simulink model "CheckFingerFunction"  (R2024a)
settings: Solver=VariableStepAuto  StartTime=0.0  StopTime=0.32  FixedStep=0.001  MaxStep=0.05  RelTol=1e-3
values from neighbouring files (symbols this model uses):
  CollisionOpacity = 0.1    [InitTestParams.m]
  g = 9.81    [InitTestParams.m]
  MotorTorque = 0.4    [InitTestParams.m]
undefined symbols (not defined in the file or in its folder): Ball, S1, S2, S3, X, Y, Z
libraries: sm_lib x404, nesl_utility x200
(part 2 of 8)

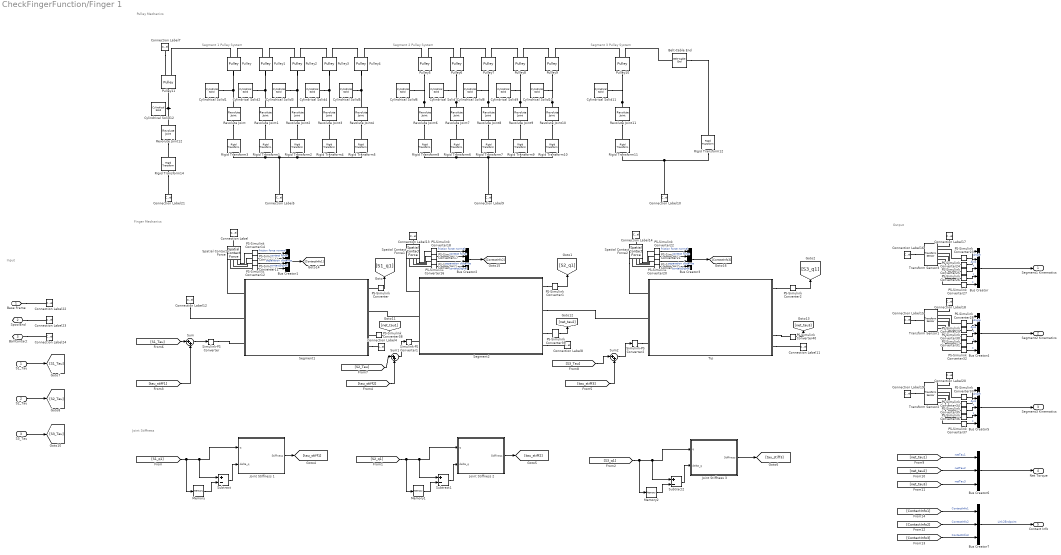
== system CheckFingerFunction/Finger 1 ==
  note: Output
  note: Input
  note: Pulley Mechanics
  note: Finger Mechanics
  note: Joint Stiffness
  note: Segment 1 Pulley System
  note: Segment 2 Pulley System
  note: Segment 3 Pulley System
  S1_Tau : Inport
  S2_Tau : Inport  Port=2
  S3_Tau : Inport  Port=3
  Belt-Cable End : sm_lib/Belts and Cables/Belt-Cable End
  Bus Creator : BusCreator  Inputs=5
  Bus Creator1 : BusCreator  Inputs=4
  Bus Creator2 : BusCreator  Inputs=4
  Bus Creator3 : BusCreator  Inputs=4
  Bus Creator4 : BusCreator  Inputs=5
  Bus Creator5 : BusCreator  Inputs=5
  Bus Creator6 : BusCreator  Inputs=3
  Bus Creator7 : BusCreator  Inputs=3
  Connection Label{,13..14,24} (4 alike) : ConnectionLabel  Label=BallContact
  Connection Label10 : ConnectionLabel  Label=PulleyFrame3
  Connection Label11 : ConnectionLabel  Label=PulleyFrame3
  Connection Label{12,15..16,19,21..22} (6 alike) : ConnectionLabel  Label=BaseFrame
  Connection Label17 : ConnectionLabel  Label=PulleyFrame1
  Connection Label18 : ConnectionLabel  Label=PulleyFrame2
  Connection Label20 : ConnectionLabel  Label=PulleyFrame3
  Connection Label23 : ConnectionLabel  Label=SpoolEnd
  Connection Label4 : ConnectionLabel  Label=PulleyFrame1
  Connection Label5 : ConnectionLabel  Label=PulleyFrame1
  Connection Label7 : ConnectionLabel  Label=SpoolEnd
  Connection Label8 : ConnectionLabel  Label=PulleyFrame2
  Connection Label9 : ConnectionLabel  Label=PulleyFrame2
  Cylindrical Solid{1..12} (12 alike) : sm_lib/Body Elements/Cylindrical Solid  CylinderRadius=1  CylinderRadiusUnits=mm  CylinderLength=1  CylinderLengthUnits=mm  ExportEntireGeometry=off  InertiaType=CalculateFromGeometry  BasedOnType=Density  Density=1000  DensityUnits=kg/m^3  Mass=1  MassUnits=kg  CenterOfMass=[0 0 0]  CenterOfMassUnits=m  MomentsOfInertia=[1 1 1]  MomentsOfInertiaUnits=kg*m^2  ProductsOfInertia=[0 0 0]  ProductsOfInertiaUnits=kg*m^2  GraphicType=FromGeometry  MarkerShape=Sphere  MarkerSize=10  GraphicVisPropType=SimpleVisualProperties  GraphicDiffuseColor=[0.5 0.5 0.5]  GraphicOpacity=1.0  GraphicSpecularColor=[0.5 0.5 0.5 1.0]  GraphicAmbientColor=[0.15 0.15 0.15 1.0]  GraphicEmissiveColor=[0.0 0.0 0.0 1.0]  GraphicShininess=75  DoExposeReferenceFrame=on  SerializedFrames=<Frames/>
  Joint Stiffness 1 : MATLAB Function  TreatAsAtomicUnit=on  mask{tau_s=0, DynamicStiffness=0}
  Joint Stiffness 2 : MATLAB Function  TreatAsAtomicUnit=on  mask{tau_s=S2.tau_s, DynamicStiffness=S2.K}
  Joint Stiffness 3 : MATLAB Function  TreatAsAtomicUnit=on  mask{tau_s=S3.tau_s, DynamicStiffness=S3.K}
  Memory : Memory
  Memory1 : Memory
  Memory2 : Memory
  PS-Simulink Converter{,1..2,11..22,38..40} (18 alike) : nesl_utility/PS-Simulink Converter  PhysicalDomain=network_engine_domain  SubClassName=ps_output  LeftPortType=input  RightPortType=output  PseudoPeriodic=off  Frequencies=[]  VectorFormat=inherit  Unit=inherit  AffineConversion=off
  PS-Simulink Converter{23..37} (15 alike) : nesl_utility/PS-Simulink Converter  PhysicalDomain=network_engine_domain  SubClassName=ps_output  LeftPortType=input  RightPortType=output  PseudoPeriodic=off  Frequencies=[]  VectorFormat=1-D array  Unit=inherit  AffineConversion=off
  Pulley{,1..11} (12 alike) : sm_lib/Belts and Cables/Pulley  PitchRadius=0.001  PitchRadiusUnits=mm  InitialWrapAngleLowerBound=0.0  InitialWrapAngleLowerBoundUnits=deg  SenseWrapAngle=off  SensePulleyAngleA=off  SensePulleyAngleB=off  SenseFleetAngleA=off  SenseFleetAngleB=off
  Revolute Joint{,1..4,6..12} (12 alike) : sm_lib/Joints/Revolute Joint  JointMode=Normal  CompositeWrenchDir=FollowerOnBase  CompositeWrenchFrame=BaseFrame  SenseConstraintForce=off  SenseConstraintTorque=off  SenseTotalForce=off  SenseTotalTorque=off  PositionTargetSpecify=off  PositionTargetPriority=High  PositionTargetValue=0  PositionTargetValueUnits=deg  VelocityTargetSpecify=off  VelocityTargetPriority=High  VelocityTargetValue=0  VelocityTargetValueUnits=deg/s  EquilibriumPosition=0  EquilibriumPositionUnits=deg  SpringStiffness=0  SpringStiffnessUnits=N*m/deg  DampingCoefficient=0  DampingCoefficientUnits=N*m/(deg/s)  LowerLimitSpecify=off  LowerLimitBound=-90  LowerLimitBoundUnits=deg  LowerLimitStiffness=1e4  LowerLimitStiffnessUnits=N*m/deg  LowerLimitDamping=10  LowerLimitDampingUnits=N*m/(deg/s)  LowerLimitTransitionRegionWidth=0.1  LowerLimitTransitionRegionWidthUnits=deg  UpperLimitSpecify=off  UpperLimitBound=90  UpperLimitBoundUnits=deg  UpperLimitStiffness=1e4  UpperLimitStiffnessUnits=N*m/deg  UpperLimitDamping=10  UpperLimitDampingUnits=N*m/(deg/s)  UpperLimitTransitionRegionWidth=0.1  UpperLimitTransitionRegionWidthUnits=deg  TorqueActuationMode=NoTorque  MotionActuationMode=ComputedMotion  SensePosition=off  SenseVelocity=off  SenseAcceleration=off  SenseTorqueForce=off  SenseLowerLimitTorqueForce=off  SenseUpperLimitTorqueForce=off
  Rigid Transform1 : sm_lib/Frames and Transforms/Rigid Transform  RotationMethod=None  FollAlignAxisA=+Z  BaseAlignAxisA=+Z  FollAlignAxisB=+X  BaseAlignAxisB=+X  RotationStandardAxis=+Z  RotationAngle=0  RotationAngleUnits=deg  RotationArbitraryAxis=[0 0 1]  RotationSequenceAxes=FollowerAxes  RotationSequence=XYX  RotationSequenceAngles=[0 0 0]  RotationSequenceAnglesUnits=deg  RotationMatrix=[1 0 0; 0 1 0; 0 0 1]  Quaternion=[1 0 0 0]  TranslationMethod=Cartesian  TranslationCartesianOffset=[12.85 4 0]  TranslationCartesianOffsetUnits=mm  TranslationStandardAxis=+Z  TranslationStandardOffset=0  TranslationStandardOffsetUnits=mm  TranslationROffset=0  TranslationROffsetUnits=m  TranslationThetaOffset=0  TranslationThetaOffsetUnits=deg  TranslationZOffset=0  TranslationZOffsetUnits=m
  Rigid Transform10 : sm_lib/Frames and Transforms/Rigid Transform  RotationMethod=None  FollAlignAxisA=+Z  BaseAlignAxisA=-Z  FollAlignAxisB=+Y  BaseAlignAxisB=+Y  RotationStandardAxis=+Z  RotationAngle=0  RotationAngleUnits=deg  RotationArbitraryAxis=[0 0 1]  RotationSequenceAxes=FollowerAxes  RotationSequence=XYX  RotationSequenceAngles=[0 0 0]  RotationSequenceAnglesUnits=deg  RotationMatrix=[1 0 0; 0 1 0; 0 0 1]  Quaternion=[1 0 0 0]  TranslationMethod=Cartesian  TranslationCartesianOffset=[30 10 0]  TranslationCartesianOffsetUnits=mm  TranslationStandardAxis=+Z  TranslationStandardOffset=0  TranslationStandardOffsetUnits=mm  TranslationROffset=0  TranslationROffsetUnits=m  TranslationThetaOffset=0  TranslationThetaOffsetUnits=deg  TranslationZOffset=0  TranslationZOffsetUnits=m
  Rigid Transform11 : sm_lib/Frames and Transforms/Rigid Transform  RotationMethod=AlignedAxes  FollAlignAxisA=-Z  BaseAlignAxisA=+Z  FollAlignAxisB=+Y  BaseAlignAxisB=+Y  RotationStandardAxis=+Z  RotationAngle=0  RotationAngleUnits=deg  RotationArbitraryAxis=[0 0 1]  RotationSequenceAxes=FollowerAxes  RotationSequence=XYX  RotationSequenceAngles=[0 0 0]  RotationSequenceAnglesUnits=deg  RotationMatrix=[1 0 0; 0 1 0; 0 0 1]  Quaternion=[1 0 0 0]  TranslationMethod=Cartesian  TranslationCartesianOffset=[14.34 3.5 0]  TranslationCartesianOffsetUnits=mm  TranslationStandardAxis=+Z  TranslationStandardOffset=0  TranslationStandardOffsetUnits=mm  TranslationROffset=0  TranslationROffsetUnits=m  TranslationThetaOffset=0  TranslationThetaOffsetUnits=deg  TranslationZOffset=0  TranslationZOffsetUnits=m
  Rigid Transform12 : sm_lib/Frames and Transforms/Rigid Transform  RotationMethod=None  FollAlignAxisA=-Z  BaseAlignAxisA=+Z  FollAlignAxisB=+Y  BaseAlignAxisB=+Y  RotationStandardAxis=+Z  RotationAngle=0  RotationAngleUnits=deg  RotationArbitraryAxis=[0 0 1]  RotationSequenceAxes=FollowerAxes  RotationSequence=XYX  RotationSequenceAngles=[0 0 0]  RotationSequenceAnglesUnits=deg  RotationMatrix=[1 0 0; 0 1 0; 0 0 1]  Quaternion=[1 0 0 0]  TranslationMethod=Cartesian  TranslationCartesianOffset=[35 -2.96 0]  TranslationCartesianOffsetUnits=mm  TranslationStandardAxis=+Z  TranslationStandardOffset=0  TranslationStandardOffsetUnits=mm  TranslationROffset=0  TranslationROffsetUnits=m  TranslationThetaOffset=0  TranslationThetaOffsetUnits=deg  TranslationZOffset=0  TranslationZOffsetUnits=m
  Rigid Transform14 : sm_lib/Frames and Transforms/Rigid Transform  RotationMethod=None  FollAlignAxisA=-Z  BaseAlignAxisA=+Z  FollAlignAxisB=+Y  BaseAlignAxisB=+Y  RotationStandardAxis=+Z  RotationAngle=0  RotationAngleUnits=deg  RotationArbitraryAxis=[0 0 1]  RotationSequenceAxes=FollowerAxes  RotationSequence=XYX  RotationSequenceAngles=[0 0 0]  RotationSequenceAnglesUnits=deg  RotationMatrix=[1 0 0; 0 1 0; 0 0 1]  Quaternion=[1 0 0 0]  TranslationMethod=Cartesian  TranslationCartesianOffset=[-13.36 -5 0]  TranslationCartesianOffsetUnits=mm  TranslationStandardAxis=+Z  TranslationStandardOffset=0  TranslationStandardOffsetUnits=mm  TranslationROffset=0  TranslationROffsetUnits=m  TranslationThetaOffset=0  TranslationThetaOffsetUnits=deg  TranslationZOffset=0  TranslationZOffsetUnits=m
  Rigid Transform2 : sm_lib/Frames and Transforms/Rigid Transform  RotationMethod=None  FollAlignAxisA=+Z  BaseAlignAxisA=+Z  FollAlignAxisB=+X  BaseAlignAxisB=+X  RotationStandardAxis=+Z  RotationAngle=0  RotationAngleUnits=deg  RotationArbitraryAxis=[0 0 1]  RotationSequenceAxes=FollowerAxes  RotationSequence=XYX  RotationSequenceAngles=[0 0 0]  RotationSequenceAnglesUnits=deg  RotationMatrix=[1 0 0; 0 1 0; 0 0 1]  Quaternion=[1 0 0 0]  TranslationMethod=Cartesian  TranslationCartesianOffset=[16.25 4 0]  TranslationCartesianOffsetUnits=mm  TranslationStandardAxis=+Z  TranslationStandardOffset=0  TranslationStandardOffsetUnits=mm  TranslationROffset=0  TranslationROffsetUnits=m  TranslationThetaOffset=0  TranslationThetaOffsetUnits=deg  TranslationZOffset=0  TranslationZOffsetUnits=m
  Rigid Transform3 : sm_lib/Frames and Transforms/Rigid Transform  RotationMethod=AlignedAxes  FollAlignAxisA=-Z  BaseAlignAxisA=+Z  FollAlignAxisB=+Y  BaseAlignAxisB=+Y  RotationStandardAxis=+Z  RotationAngle=0  RotationAngleUnits=deg  RotationArbitraryAxis=[0 0 1]  RotationSequenceAxes=FollowerAxes  RotationSequence=XYX  RotationSequenceAngles=[0 0 0]  RotationSequenceAnglesUnits=deg  RotationMatrix=[1 0 0; 0 1 0; 0 0 1]  Quaternion=[1 0 0 0]  TranslationMethod=Cartesian  TranslationCartesianOffset=[8.85 7.5 0]  TranslationCartesianOffsetUnits=mm  TranslationStandardAxis=+Z  TranslationStandardOffset=0  TranslationStandardOffsetUnits=mm  TranslationROffset=0  TranslationROffsetUnits=m  TranslationThetaOffset=0  TranslationThetaOffsetUnits=deg  TranslationZOffset=0  TranslationZOffsetUnits=m
  Rigid Transform4 : sm_lib/Frames and Transforms/Rigid Transform  RotationMethod=AlignedAxes  FollAlignAxisA=+Z  BaseAlignAxisA=-Z  FollAlignAxisB=+Y  BaseAlignAxisB=+Y  RotationStandardAxis=+Z  RotationAngle=0  RotationAngleUnits=deg  RotationArbitraryAxis=[0 0 1]  RotationSequenceAxes=FollowerAxes  RotationSequence=XYX  RotationSequenceAngles=[0 0 0]  RotationSequenceAnglesUnits=deg  RotationMatrix=[1 0 0; 0 1 0; 0 0 1]  Quaternion=[1 0 0 0]  TranslationMethod=Cartesian  TranslationCartesianOffset=[21.1 7.5 0]  TranslationCartesianOffsetUnits=mm  TranslationStandardAxis=+Z  TranslationStandardOffset=0  TranslationStandardOffsetUnits=mm  TranslationROffset=0  TranslationROffsetUnits=m  TranslationThetaOffset=0  TranslationThetaOffsetUnits=deg  TranslationZOffset=0  TranslationZOffsetUnits=m
  Rigid Transform5 : sm_lib/Frames and Transforms/Rigid Transform  RotationMethod=None  FollAlignAxisA=+Z  BaseAlignAxisA=-Z  FollAlignAxisB=+Y  BaseAlignAxisB=+Y  RotationStandardAxis=+Z  RotationAngle=0  RotationAngleUnits=deg  RotationArbitraryAxis=[0 0 1]  RotationSequenceAxes=FollowerAxes  RotationSequence=XYX  RotationSequenceAngles=[0 0 0]  RotationSequenceAnglesUnits=deg  RotationMatrix=[1 0 0; 0 1 0; 0 0 1]  Quaternion=[1 0 0 0]  TranslationMethod=Cartesian  TranslationCartesianOffset=[30 10 0]  TranslationCartesianOffsetUnits=mm  TranslationStandardAxis=+Z  TranslationStandardOffset=0  TranslationStandardOffsetUnits=mm  TranslationROffset=0  TranslationROffsetUnits=m  TranslationThetaOffset=0  TranslationThetaOffsetUnits=deg  TranslationZOffset=0  TranslationZOffsetUnits=m
  Rigid Transform6 : sm_lib/Frames and Transforms/Rigid Transform  RotationMethod=None  FollAlignAxisA=+Z  BaseAlignAxisA=+Z  FollAlignAxisB=+X  BaseAlignAxisB=+X  RotationStandardAxis=+Z  RotationAngle=0  RotationAngleUnits=deg  RotationArbitraryAxis=[0 0 1]  RotationSequenceAxes=FollowerAxes  RotationSequence=XYX  RotationSequenceAngles=[0 0 0]  RotationSequenceAnglesUnits=deg  RotationMatrix=[1 0 0; 0 1 0; 0 0 1]  Quaternion=[1 0 0 0]  TranslationMethod=Cartesian  TranslationCartesianOffset=[12.85 4 0]  TranslationCartesianOffsetUnits=mm  TranslationStandardAxis=+Z  TranslationStandardOffset=0  TranslationStandardOffsetUnits=mm  TranslationROffset=0  TranslationROffsetUnits=m  TranslationThetaOffset=0  TranslationThetaOffsetUnits=deg  TranslationZOffset=0  TranslationZOffsetUnits=m
  Rigid Transform7 : sm_lib/Frames and Transforms/Rigid Transform  RotationMethod=None  FollAlignAxisA=+Z  BaseAlignAxisA=+Z  FollAlignAxisB=+X  BaseAlignAxisB=+X  RotationStandardAxis=+Z  RotationAngle=0  RotationAngleUnits=deg  RotationArbitraryAxis=[0 0 1]  RotationSequenceAxes=FollowerAxes  RotationSequence=XYX  RotationSequenceAngles=[0 0 0]  RotationSequenceAnglesUnits=deg  RotationMatrix=[1 0 0; 0 1 0; 0 0 1]  Quaternion=[1 0 0 0]  TranslationMethod=Cartesian  TranslationCartesianOffset=[16.25 4 0]  TranslationCartesianOffsetUnits=mm  TranslationStandardAxis=+Z  TranslationStandardOffset=0  TranslationStandardOffsetUnits=mm  TranslationROffset=0  TranslationROffsetUnits=m  TranslationThetaOffset=0  TranslationThetaOffsetUnits=deg  TranslationZOffset=0  TranslationZOffsetUnits=m
  Rigid Transform8 : sm_lib/Frames and Transforms/Rigid Transform  RotationMethod=AlignedAxes  FollAlignAxisA=-Z  BaseAlignAxisA=+Z  FollAlignAxisB=+Y  BaseAlignAxisB=+Y  RotationStandardAxis=+Z  RotationAngle=0  RotationAngleUnits=deg  RotationArbitraryAxis=[0 0 1]  RotationSequenceAxes=FollowerAxes  RotationSequence=XYX  RotationSequenceAngles=[0 0 0]  RotationSequenceAnglesUnits=deg  RotationMatrix=[1 0 0; 0 1 0; 0 0 1]  Quaternion=[1 0 0 0]  TranslationMethod=Cartesian  TranslationCartesianOffset=[8.85 7.5 0]  TranslationCartesianOffsetUnits=mm  TranslationStandardAxis=+Z  TranslationStandardOffset=0  TranslationStandardOffsetUnits=mm  TranslationROffset=0  TranslationROffsetUnits=m  TranslationThetaOffset=0  TranslationThetaOffsetUnits=deg  TranslationZOffset=0  TranslationZOffsetUnits=m
  Rigid Transform9 : sm_lib/Frames and Transforms/Rigid Transform  RotationMethod=AlignedAxes  FollAlignAxisA=+Z  BaseAlignAxisA=-Z  FollAlignAxisB=+Y  BaseAlignAxisB=+Y  RotationStandardAxis=+Z  RotationAngle=0  RotationAngleUnits=deg  RotationArbitraryAxis=[0 0 1]  RotationSequenceAxes=FollowerAxes  RotationSequence=XYX  RotationSequenceAngles=[0 0 0]  RotationSequenceAnglesUnits=deg  RotationMatrix=[1 0 0; 0 1 0; 0 0 1]  Quaternion=[1 0 0 0]  TranslationMethod=Cartesian  TranslationCartesianOffset=[21.1 7.5 0]  TranslationCartesianOffsetUnits=mm  TranslationStandardAxis=+Z  TranslationStandardOffset=0  TranslationStandardOffsetUnits=mm  TranslationROffset=0  TranslationROffsetUnits=m  TranslationThetaOffset=0  TranslationThetaOffsetUnits=deg  TranslationZOffset=0  TranslationZOffsetUnits=m
  Segment1 : Subsystem  mask{JointDamping=S1.JointDamping, upperLimit=S1.upperLimit, lowerLimit=S1.lowerLimit, InitAngle=S1.InitAngle, Axle2Axle_mm=S1.Axle2AxleDist_mm, CollisionOpacity=CollisionOpacity}
      mask prompts: JointDamping "Joint Damping (N s/m/rad)"; upperLimit "Upper Limit (deg)"; lowerLimit "Lower Limit (deg)"; InitAngle "Initial Angle (deg)"; Axle2Axle_mm "Axle to Axle distance (mm)"; CollisionOpacity "Collision Opacity"
  Segment2 : Subsystem  mask{JointDamping=S1.JointDamping, upperLimit=S1.upperLimit, lowerLimit=S1.lowerLimit, InitAngle=S1.InitAngle, Axle2Axle_mm=S1.Axle2AxleDist_mm, CollisionOpacity=CollisionOpacity}
      mask prompts: JointDamping "Joint Damping (N s/m/rad)"; upperLimit "Upper Limit (deg)"; lowerLimit "Lower Limit (deg)"; InitAngle "Initial Angle (deg)"; Axle2Axle_mm "Axle to Axle distance (mm)"; CollisionOpacity "Collision Opacity"
  Simulink-PS Converter : nesl_utility/Simulink-PS Converter  PhysicalDomain=network_engine_domain  SubClassName=ps_input  LeftPortType=input  RightPortType=output  PseudoPeriodic=off  Frequencies=[]  NoiseDistribution=none  NoiseParameters=[]  Unit=1  AffineConversion=off  FilteringAndDerivatives=provide  SimscapeFilterOrder=1  InputFilterTimeConstant=0.001  UdotUserProvided=0
  Simulink-PS Converter1 : nesl_utility/Simulink-PS Converter  PhysicalDomain=network_engine_domain  SubClassName=ps_input  LeftPortType=input  RightPortType=output  PseudoPeriodic=off  Frequencies=[]  NoiseDistribution=none  NoiseParameters=[]  Unit=1  AffineConversion=off  FilteringAndDerivatives=provide  SimscapeFilterOrder=1  InputFilterTimeConstant=0.001  UdotUserProvided=0
  Simulink-PS Converter2 : nesl_utility/Simulink-PS Converter  PhysicalDomain=network_engine_domain  SubClassName=ps_input  LeftPortType=input  RightPortType=output  PseudoPeriodic=off  Frequencies=[]  NoiseDistribution=none  NoiseParameters=[]  Unit=1  AffineConversion=off  FilteringAndDerivatives=provide  SimscapeFilterOrder=1  InputFilterTimeConstant=0.001  UdotUserProvided=0
  Spatial Contact Force : sm_lib/Forces and Torques/Spatial Contact Force  NormalForceType=SmoothSpringDamper  NormalStiffness=S1.ContactStiffness  NormalStiffnessUnits=N/m  NormalDamping=S1.ContactDamping  NormalDampingUnits=N/(m/s)  NormalTransitionRegionWidth=1e-4  NormalTransitionRegionWidthUnits=m  FrictionType=SmoothStickSlip  CoefficientOfStaticFriction=0.5  CoefficientOfDynamicFriction=0.3  FrictionalCriticalVelocity=1e-3  FrictionalCriticalVelocityUnits=m/s  SenseContactSignal=on  SensePenetrationDepth=off  SenseSeparationDistance=on  SenseNormalForceMagnitude=on  SenseFrictionalForceMagnitude=on  SenseNormalVelocity=off  SenseTangentialVelocity=off  SenseContactBaseRotation=off  SenseContactBaseTranslation=off  SenseContactFollowerRotation=off  SenseContactFollowerTranslation=off  ZeroCrossDetectContactStartAndEnd=off
  Spatial Contact Force1 : sm_lib/Forces and Torques/Spatial Contact Force  NormalForceType=SmoothSpringDamper  NormalStiffness=S2.ContactStiffness  NormalStiffnessUnits=N/m  NormalDamping=S2.ContactDamping  NormalDampingUnits=N/(m/s)  NormalTransitionRegionWidth=1e-4  NormalTransitionRegionWidthUnits=m  FrictionType=SmoothStickSlip  CoefficientOfStaticFriction=0.5  CoefficientOfDynamicFriction=0.3  FrictionalCriticalVelocity=1e-3  FrictionalCriticalVelocityUnits=m/s  SenseContactSignal=on  SensePenetrationDepth=off  SenseSeparationDistance=on  SenseNormalForceMagnitude=on  SenseFrictionalForceMagnitude=on  SenseNormalVelocity=off  SenseTangentialVelocity=off  SenseContactBaseRotation=off  SenseContactBaseTranslation=off  SenseContactFollowerRotation=off  SenseContactFollowerTranslation=off  ZeroCrossDetectContactStartAndEnd=off
  Spatial Contact Force2 : sm_lib/Forces and Torques/Spatial Contact Force  NormalForceType=SmoothSpringDamper  NormalStiffness=S3.ContactStiffness  NormalStiffnessUnits=N/m  NormalDamping=S3.ContactDamping  NormalDampingUnits=N/(m/s)  NormalTransitionRegionWidth=1e-4  NormalTransitionRegionWidthUnits=m  FrictionType=SmoothStickSlip  CoefficientOfStaticFriction=0.5  CoefficientOfDynamicFriction=0.3  FrictionalCriticalVelocity=1e-3  FrictionalCriticalVelocityUnits=m/s  SenseContactSignal=on  SensePenetrationDepth=off  SenseSeparationDistance=on  SenseNormalForceMagnitude=on  SenseFrictionalForceMagnitude=on  SenseNormalVelocity=off  SenseTangentialVelocity=off  SenseContactBaseRotation=off  SenseContactBaseTranslation=off  SenseContactFollowerRotation=off  SenseContactFollowerTranslation=off  ZeroCrossDetectContactStartAndEnd=off
  Subtract : Sum  Inputs=+-
  Subtract1 : Sum  Inputs=+-
  Subtract2 : Sum  Inputs=+-
  Sum : Sum  Inputs=|++
  Sum1 : Sum  Inputs=|++
  Sum2 : Sum  Inputs=|++
  Tip : Subsystem  mask{JointDamping=S3.JointDamping, upperLimit=S3.upperLimit, lowerLimit=S3.lowerLimit, InitAngle=S3.InitAngle, Axle2Axle_mm=S3.Axle2AxleDist_mm, CollisionOpacity=CollisionOpacity}
      mask prompts: JointDamping "Joint Damping (N s/m/rad)"; upperLimit "Upper Limit (deg)"; lowerLimit "Lower Limit (deg)"; InitAngle "Initial Angle (deg)"; Axle2Axle_mm "Axle to Axle distance (mm)"; CollisionOpacity "Collision Opacity"
  Transform Sensor1 : sm_lib/Frames and Transforms/Transform Sensor  MeasurementFrame=World  RotationSequence=XYX  SenseAngle=on  SenseAxis=on  SenseQ=off  SenseR=off  SenseRotationSequence=off  SenseOmegaX=off  SenseOmegaY=off  SenseOmegaZ=off  SenseOmega=off  SenseQDot=off  SenseRDot=off  SenseRotationSequenceDot=off  SenseAlphaX=off  SenseAlphaY=off  SenseAlphaZ=off  SenseAlpha=off  SenseQDDot=off  SenseRDDot=off  SenseX=on  SenseY=on  SenseZ=on  SenseXYZ=off  SenseRad=off  SenseAzim=off  SenseDist=off  SenseInc=off  SenseXDot=off  SenseYDot=off  SenseZDot=off  SenseXYZDot=off  SenseRadDot=off  SenseAzimDot=off  SenseDistDot=off  SenseIncDot=off  SenseXDDot=off  SenseYDDot=off  SenseZDDot=off  SenseXYZDDot=off  SenseRadDDot=off  SenseAzimDDot=off  SenseDistDDot=off  SenseIncDDot=off
  Transform Sensor2 : sm_lib/Frames and Transforms/Transform Sensor  MeasurementFrame=World  RotationSequence=XYX  SenseAngle=on  SenseAxis=on  SenseQ=off  SenseR=off  SenseRotationSequence=off  SenseOmegaX=off  SenseOmegaY=off  SenseOmegaZ=off  SenseOmega=off  SenseQDot=off  SenseRDot=off  SenseRotationSequenceDot=off  SenseAlphaX=off  SenseAlphaY=off  SenseAlphaZ=off  SenseAlpha=off  SenseQDDot=off  SenseRDDot=off  SenseX=on  SenseY=on  SenseZ=on  SenseXYZ=off  SenseRad=off  SenseAzim=off  SenseDist=off  SenseInc=off  SenseXDot=off  SenseYDot=off  SenseZDot=off  SenseXYZDot=off  SenseRadDot=off  SenseAzimDot=off  SenseDistDot=off  SenseIncDot=off  SenseXDDot=off  SenseYDDot=off  SenseZDDot=off  SenseXYZDDot=off  SenseRadDDot=off  SenseAzimDDot=off  SenseDistDDot=off  SenseIncDDot=off
  Transform Sensor3 : sm_lib/Frames and Transforms/Transform Sensor  MeasurementFrame=World  RotationSequence=XYX  SenseAngle=on  SenseAxis=on  SenseQ=off  SenseR=off  SenseRotationSequence=off  SenseOmegaX=off  SenseOmegaY=off  SenseOmegaZ=off  SenseOmega=off  SenseQDot=off  SenseRDot=off  SenseRotationSequenceDot=off  SenseAlphaX=off  SenseAlphaY=off  SenseAlphaZ=off  SenseAlpha=off  SenseQDDot=off  SenseRDDot=off  SenseX=on  SenseY=on  SenseZ=on  SenseXYZ=off  SenseRad=off  SenseAzim=off  SenseDist=off  SenseInc=off  SenseXDot=off  SenseYDot=off  SenseZDot=off  SenseXYZDot=off  SenseRadDot=off  SenseAzimDot=off  SenseDistDot=off  SenseIncDot=off  SenseXDDot=off  SenseYDDot=off  SenseZDDot=off  SenseXYZDDot=off  SenseRadDDot=off  SenseAzimDDot=off  SenseDistDDot=off  SenseIncDDot=off
  Base Frame : PMIOPort  Side=Left
  SpoolEnd : PMIOPort  Port=2  Side=Left
  BallContact : PMIOPort  Port=3  Side=Left
  Segment1 Kinematics : Outport
  Segment2 Kinematics : Outport  Port=2
  Segment3 Kinematics : Outport  Port=3
  Net Torque : Outport  Port=4
  Contact Info : Outport  Port=5
  wires:
  PS-Simulink Converter33/1 -> Bus Creator5/1  "Angle"
  Memory2/1 -> Subtract2/2
  [tau_stiff1] -> Sum/2
  [S2_q1] -> Subtract1/1, Joint Stiffness 2/1(q), Memory1/1
  PS-Simulink Converter26/1 -> Bus Creator/4  "y"
  PS-Simulink Converter1/1 -> [S2_q1]
  PS-Simulink Converter27/1 -> Bus Creator/5  "z"
  PS-Simulink Converter18/1 -> Bus Creator2/1  "friction force normal"
  [S1_q1] -> Subtract/1, Joint Stiffness 1/1(q), Memory/1
  Subtract1/1 -> Joint Stiffness 2/2(delta_q)
  Subtract2/1 -> Joint Stiffness 3/2(delta_q)
  Subtract/1 -> Joint Stiffness 1/2(delta_q)
  [S2_Tau] -> Sum1/1
  Memory/1 -> Subtract/2
  PS-Simulink Converter14/1 -> Bus Creator1/1  "friction force normal"
  PS-Simulink Converter11/1 -> Bus Creator1/4  "contactSignal"
  PS-Simulink Converter35/1 -> Bus Creator5/3  "x"
  PS-Simulink Converter16/1 -> Bus Creator2/3  "separation distance"
  Joint Stiffness 3/1(Stiffness) -> [tau_stiff3]
  PS-Simulink Converter31/1 -> Bus Creator4/4  "y"
  PS-Simulink Converter28/1 -> Bus Creator4/1  "Angle"
  [S3_q1] -> Subtract2/1, Joint Stiffness 3/1(q), Memory2/1
  Bus Creator5/1 -> Segment3 Kinematics/1
  S3_Tau/1 -> [S3_Tau]
  Memory1/1 -> Subtract1/2
  PS-Simulink Converter15/1 -> Bus Creator2/4  "contactSignal"
  PS-Simulink Converter2/1 -> [S3_q1]
  Bus Creator2/1 -> [ContactInfo2]
  [S3_Tau] -> Sum2/1
  Bus Creator/1 -> Segment1 Kinematics/1
  PS-Simulink Converter/1 -> [S1_q1]
  Sum1/1 -> Simulink-PS Converter1/1
  PS-Simulink Converter24/1 -> Bus Creator/2  "Axis"
  PS-Simulink Converter25/1 -> Bus Creator/3  "x"
  S2_Tau/1 -> [S2_Tau]
  PS-Simulink Converter29/1 -> Bus Creator4/2  "Axis"
  [net_tau2] -> Bus Creator6/2  "netTau2"
  PS-Simulink Converter23/1 -> Bus Creator/1  "Angle"
  PS-Simulink Converter34/1 -> Bus Creator5/2  "Axis"
  S1_Tau/1 -> [S1_Tau]
  [S1_Tau] -> Sum/1
  Joint Stiffness 2/1(Stiffness) -> [tau_stiff2]
  PS-Simulink Converter32/1 -> Bus Creator4/5  "z"
  Bus Creator4/1 -> Segment2 Kinematics/1
  PS-Simulink Converter40/1 -> [net_tau3]
  Bus Creator7/1 -> Contact Info/1  "Link2Endpoint"
  PS-Simulink Converter20/1 -> Bus Creator3/3  "separation distance"
  PS-Simulink Converter19/1 -> Bus Creator3/4  "contactSignal"
  PS-Simulink Converter22/1 -> Bus Creator3/1  "friction force normal"
  PS-Simulink Converter21/1 -> Bus Creator3/2  "contact force"
  Joint Stiffness 1/1(Stiffness) -> [tau_stiff1]
  PS-Simulink Converter12/1 -> Bus Creator1/3  "separation distance"
  [tau_stiff3] -> Sum2/2
  PS-Simulink Converter30/1 -> Bus Creator4/3  "x"
  Sum/1 -> Simulink-PS Converter/1
  [tau_stiff2] -> Sum1/2
  Sum2/1 -> Simulink-PS Converter2/1
  Bus Creator3/1 -> [ContactInfo3]
  PS-Simulink Converter13/1 -> Bus Creator1/2  "contact force"
  [net_tau3] -> Bus Creator6/3  "netTau3"
  PS-Simulink Converter36/1 -> Bus Creator5/4  "y"
  PS-Simulink Converter37/1 -> Bus Creator5/5  "z"
  [net_tau1] -> Bus Creator6/1  "netTau1"
  PS-Simulink Converter38/1 -> [net_tau1]
  PS-Simulink Converter17/1 -> Bus Creator2/2  "contact force"
  Bus Creator1/1 -> [ContactInfo1]
  [ContactInfo3] -> Bus Creator7/3  "ContactInfo3"
  [ContactInfo1] -> Bus Creator7/1  "ContactInfo1"
  [ContactInfo2] -> Bus Creator7/2  "ContactInfo2"
  PS-Simulink Converter39/1 -> [net_tau2]
  Bus Creator6/1 -> Net Torque/1
  connections:
  Revolute Joint11/RConn1 -- Cylindrical Solid11/RConn1 -- Pulley10/LConn1
  Pulley7/RConn2 -- Pulley8/RConn1
  Simulink-PS Converter/RConn1 -- Segment1/LConn3
  PS-Simulink Converter11/LConn1 -- Spatial Contact Force/RConn2
  PS-Simulink Converter26/LConn1 -- Transform Sensor3/RConn5
  Pulley/LConn1 -- Cylindrical Solid1/RConn1 -- Revolute Joint/RConn1
  Connection Label13/LConn1 -- Spatial Contact Force1/LConn1
  Pulley8/RConn2 -- Pulley9/RConn1
  PS-Simulink Converter19/LConn1 -- Spatial Contact Force2/RConn2
  Segment2/LConn1 -- Spatial Contact Force1/RConn1
  Pulley3/RConn2 -- Pulley4/RConn1
  PS-Simulink Converter16/LConn1 -- Spatial Contact Force1/RConn3
  Spatial Contact Force2/LConn1 -- Connection Label14/LConn1
  Segment2/RConn6 -- Connection Label8/LConn1
  Belt-Cable End/RConn1 -- Pulley10/RConn2
  Connection Label17/LConn1 -- Transform Sensor3/RConn1
  Pulley3/LConn1 -- Cylindrical Solid4/RConn1 -- Revolute Joint3/RConn1
  Revolute Joint7/RConn1 -- Cylindrical Solid7/RConn1 -- Pulley6/LConn1
  Base Frame/RConn1 -- Connection Label22/LConn1
  Pulley6/RConn2 -- Pulley7/RConn1
  Spatial Contact Force/LConn1 -- Connection Label/LConn1
  PS-Simulink Converter12/LConn1 -- Spatial Contact Force/RConn3
  Pulley2/LConn1 -- Cylindrical Solid3/RConn1 -- Revolute Joint2/RConn1
  Tip/RConn1 -- PS-Simulink Converter2/LConn1
  Spatial Contact Force1/RConn5 -- PS-Simulink Converter18/LConn1
  Revolute Joint3/LConn1 -- Rigid Transform4/RConn1
  PS-Simulink Converter/LConn1 -- Segment1/RConn1
  Rigid Transform12/LConn1 -- Connection Label10/LConn1 -- Rigid Transform11/LConn1
  Rigid Transform3/LConn1 -- Connection Label5/LConn1 -- Rigid Transform5/LConn1 -- Rigid Transform4/LConn1 -- Rigid Transform2/LConn1 -- Rigid Transform1/LConn1
  Rigid Transform6/LConn1 -- Rigid Transform8/LConn1 -- Rigid Transform10/LConn1 -- Rigid Transform9/LConn1 -- Connection Label9/LConn1 -- Rigid Transform7/LConn1
  PS-Simulink Converter24/LConn1 -- Transform Sensor3/RConn3
  PS-Simulink Converter30/LConn1 -- Transform Sensor1/RConn4
  PS-Simulink Converter29/LConn1 -- Transform Sensor1/RConn3
  Segment2/RConn3 -- Tip/LConn2
  Revolute Joint9/LConn1 -- Rigid Transform9/RConn1
  PS-Simulink Converter31/LConn1 -- Transform Sensor1/RConn5
  Revolute Joint11/LConn1 -- Rigid Transform11/RConn1
  Simulink-PS Converter2/RConn1 -- Tip/LConn3
  Pulley1/LConn1 -- Cylindrical Solid2/RConn1 -- Revolute Joint1/RConn1
  PS-Simulink Converter35/LConn1 -- Transform Sensor2/RConn4
  Connection Label16/LConn1 -- Transform Sensor3/LConn1
  Revolute Joint8/RConn1 -- Cylindrical Solid8/RConn1 -- Pulley7/LConn1
  Revolute Joint/LConn1 -- Rigid Transform3/RConn1
  PS-Simulink Converter13/LConn1 -- Spatial Contact Force/RConn4
  Connection Label7/LConn1 -- Pulley11/RConn1
  PS-Simulink Converter20/LConn1 -- Spatial Contact Force2/RConn3
  PS-Simulink Converter23/LConn1 -- Transform Sensor3/RConn2
  Belt-Cable End/LConn1 -- Rigid Transform12/RConn1
  Connection Label18/LConn1 -- Transform Sensor1/RConn1
  PS-Simulink Converter32/LConn1 -- Transform Sensor1/RConn6
  PS-Simulink Converter27/LConn1 -- Transform Sensor3/RConn6
  Revolute Joint10/LConn1 -- Rigid Transform10/RConn1
  Connection Label15/LConn1 -- Transform Sensor1/LConn1
  PS-Simulink Converter28/LConn1 -- Transform Sensor1/RConn2
  Segment1/RConn6 -- Connection Label4/LConn1
  Rigid Transform14/LConn1 -- Connection Label21/LConn1
  PS-Simulink Converter21/LConn1 -- Spatial Contact Force2/RConn4
  Spatial Contact Force2/RConn5 -- PS-Simulink Converter22/LConn1
  PS-Simulink Converter15/LConn1 -- Spatial Contact Force1/RConn2
  Connection Label12/LConn1 -- Segment1/LConn2
  Spatial Contact Force2/RConn1 -- Tip/LConn1
  Pulley1/RConn2 -- Pulley2/RConn1
  Revolute Joint2/LConn1 -- Rigid Transform2/RConn1
  Revolute Joint4/LConn1 -- Rigid Transform5/RConn1
  Revolute Joint1/LConn1 -- Rigid Transform1/RConn1
  Segment1/LConn1 -- Spatial Contact Force/RConn1
  Revolute Joint12/LConn1 -- Rigid Transform14/RConn1
  Pulley4/LConn1 -- Cylindrical Solid5/RConn1 -- Revolute Joint4/RConn1
  Connection Label19/LConn1 -- Transform Sensor2/LConn1
  PS-Simulink Converter25/LConn1 -- Transform Sensor3/RConn4
  Pulley10/RConn1 -- Pulley9/RConn2
  Segment2/LConn2 -- Segment1/RConn3
  Revolute Joint6/RConn1 -- Cylindrical Solid6/RConn1 -- Pulley5/LConn1
  PS-Simulink Converter37/LConn1 -- Transform Sensor2/RConn6
  Revolute Joint10/RConn1 -- Cylindrical Solid10/RConn1 -- Pulley9/LConn1
  Revolute Joint7/LConn1 -- Rigid Transform6/RConn1
  Tip/RConn5 -- PS-Simulink Converter40/LConn1
  Revolute Joint9/RConn1 -- Cylindrical Solid9/RConn1 -- Pulley8/LConn1
  Revolute Joint6/LConn1 -- Rigid Transform8/RConn1
  Revolute Joint8/LConn1 -- Rigid Transform7/RConn1
  Pulley2/RConn2 -- Pulley3/RConn1
  Pulley1/RConn1 -- Pulley/RConn2
  Pulley5/RConn2 -- Pulley6/RConn1
  Segment2/LConn3 -- Simulink-PS Converter1/RConn1
  Segment2/RConn1 -- PS-Simulink Converter1/LConn1
  Pulley4/RConn2 -- Pulley5/RConn1
  Revolute Joint12/RConn1 -- Cylindrical Solid12/RConn1 -- Pulley11/LConn1
  Spatial Contact Force/RConn5 -- PS-Simulink Converter14/LConn1
  PS-Simulink Converter38/LConn1 -- Segment1/RConn5
  Tip/RConn6 -- Connection Label11/LConn1
  Connection Label20/LConn1 -- Transform Sensor2/RConn1
  PS-Simulink Converter33/LConn1 -- Transform Sensor2/RConn2
  PS-Simulink Converter34/LConn1 -- Transform Sensor2/RConn3
  PS-Simulink Converter36/LConn1 -- Transform Sensor2/RConn5
  PS-Simulink Converter17/LConn1 -- Spatial Contact Force1/RConn4
  SpoolEnd/RConn1 -- Connection Label23/LConn1
  BallContact/RConn1 -- Connection Label24/LConn1
  Pulley11/RConn2 -- Pulley/RConn1
  Segment2/RConn5 -- PS-Simulink Converter39/LConn1
